simulink model "adsl_sim"  (Simulink 6.0)
settings: Solver=ode45  SolverMode=SingleTasking  StartTime=0.0  StopTime=2  RelTol=1e-3
PreLoadFcn:
  | % variables are initialized through the Model Workspace
model workspace: external: M-Code (data not in the file)
values from neighbouring files (symbols this model uses):
  H = conv2(chCoeff',W)    [eq_computecostfcn.m]    (also in eq_costfcnconverg.m = conv2(eq.chCoeff,W))
undefined symbols (not defined in the file or in its folder): b, rsgenpoly, slcm
libraries: commdigbbndam2 x512, simulink x37, commutil2 x8, commblkcod2 x4, commsequence2 x4, commsink2 x4, commcrc2 x4, commcnvintrlv2 x2, dspxfrm3 x2, dspsrcs4 x2, dspsigattribs x1, dspmtrx3 x1
(part 2 of 5)

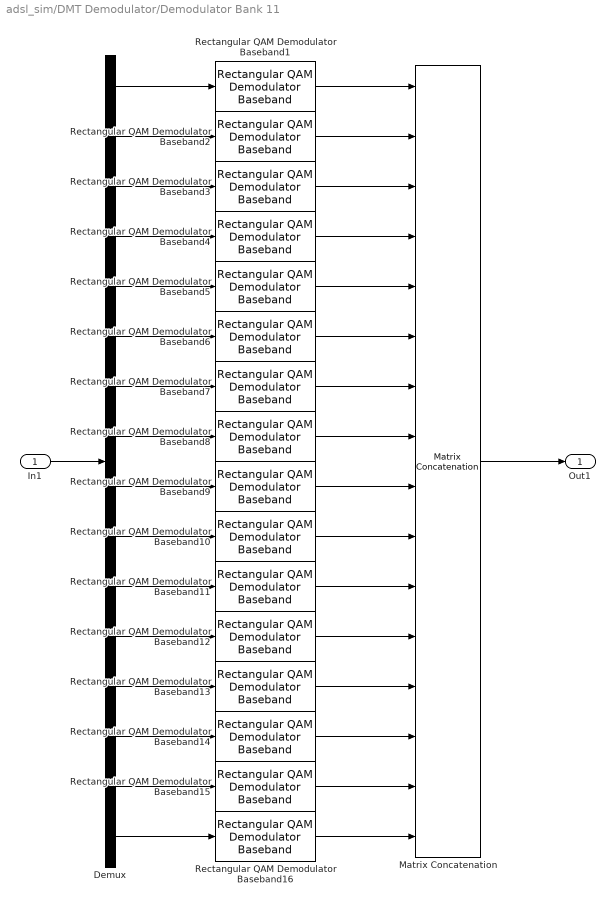
== system adsl_sim/DMT Demodulator/Demodulator Bank 11 ==
  In1 : Inport  LatchInput=off
  Demux : Demux  Outputs=16
  Matrix Concatenation : simulink/Math Operations/Matrix Concatenation  numInports=16  catMethod=Vertical
  Rectangular QAM Demodulator Baseband1 : commdigbbndam2/Rectangular QAM Demodulator Baseband  M=2^b(offset+1)  OutType=Bit  Dec=Gray  PowType=Average Power  MinDist=2  AvgPow=1  PeakPow=1  Ph=0  numSamp=1
  Rectangular QAM Demodulator Baseband10 : commdigbbndam2/Rectangular QAM Demodulator Baseband  M=2^b(offset+10)  OutType=Bit  Dec=Gray  PowType=Average Power  MinDist=2  AvgPow=1  PeakPow=1  Ph=0  numSamp=1
  Rectangular QAM Demodulator Baseband11 : commdigbbndam2/Rectangular QAM Demodulator Baseband  M=2^b(offset+11)  OutType=Bit  Dec=Gray  PowType=Average Power  MinDist=2  AvgPow=1  PeakPow=1  Ph=0  numSamp=1
  Rectangular QAM Demodulator Baseband12 : commdigbbndam2/Rectangular QAM Demodulator Baseband  M=2^b(offset+12)  OutType=Bit  Dec=Gray  PowType=Average Power  MinDist=2  AvgPow=1  PeakPow=1  Ph=0  numSamp=1
  Rectangular QAM Demodulator Baseband13 : commdigbbndam2/Rectangular QAM Demodulator Baseband  M=2^b(offset+13)  OutType=Bit  Dec=Gray  PowType=Average Power  MinDist=2  AvgPow=1  PeakPow=1  Ph=0  numSamp=1
  Rectangular QAM Demodulator Baseband14 : commdigbbndam2/Rectangular QAM Demodulator Baseband  M=2^b(offset+14)  OutType=Bit  Dec=Gray  PowType=Average Power  MinDist=2  AvgPow=1  PeakPow=1  Ph=0  numSamp=1
  Rectangular QAM Demodulator Baseband15 : commdigbbndam2/Rectangular QAM Demodulator Baseband  M=2^b(offset+15)  OutType=Bit  Dec=Gray  PowType=Average Power  MinDist=2  AvgPow=1  PeakPow=1  Ph=0  numSamp=1
  Rectangular QAM Demodulator Baseband16 : commdigbbndam2/Rectangular QAM Demodulator Baseband  M=2^b(offset+16)  OutType=Bit  Dec=Gray  PowType=Average Power  MinDist=2  AvgPow=1  PeakPow=1  Ph=0  numSamp=1
  Rectangular QAM Demodulator Baseband2 : commdigbbndam2/Rectangular QAM Demodulator Baseband  M=2^b(offset+2)  OutType=Bit  Dec=Gray  PowType=Average Power  MinDist=2  AvgPow=1  PeakPow=1  Ph=0  numSamp=1
  Rectangular QAM Demodulator Baseband3 : commdigbbndam2/Rectangular QAM Demodulator Baseband  M=2^b(offset+3)  OutType=Bit  Dec=Gray  PowType=Average Power  MinDist=2  AvgPow=1  PeakPow=1  Ph=0  numSamp=1
  Rectangular QAM Demodulator Baseband4 : commdigbbndam2/Rectangular QAM Demodulator Baseband  M=2^b(offset+4)  OutType=Bit  Dec=Gray  PowType=Average Power  MinDist=2  AvgPow=1  PeakPow=1  Ph=0  numSamp=1
  Rectangular QAM Demodulator Baseband5 : commdigbbndam2/Rectangular QAM Demodulator Baseband  M=2^b(offset+5)  OutType=Bit  Dec=Gray  PowType=Average Power  MinDist=2  AvgPow=1  PeakPow=1  Ph=0  numSamp=1
  Rectangular QAM Demodulator Baseband6 : commdigbbndam2/Rectangular QAM Demodulator Baseband  M=2^b(offset+6)  OutType=Bit  Dec=Gray  PowType=Average Power  MinDist=2  AvgPow=1  PeakPow=1  Ph=0  numSamp=1
  Rectangular QAM Demodulator Baseband7 : commdigbbndam2/Rectangular QAM Demodulator Baseband  M=2^b(offset+7)  OutType=Bit  Dec=Gray  PowType=Average Power  MinDist=2  AvgPow=1  PeakPow=1  Ph=0  numSamp=1
  Rectangular QAM Demodulator Baseband8 : commdigbbndam2/Rectangular QAM Demodulator Baseband  M=2^b(offset+8)  OutType=Bit  Dec=Gray  PowType=Average Power  MinDist=2  AvgPow=1  PeakPow=1  Ph=0  numSamp=1
  Rectangular QAM Demodulator Baseband9 : commdigbbndam2/Rectangular QAM Demodulator Baseband  M=2^b(offset+9)  OutType=Bit  Dec=Gray  PowType=Average Power  MinDist=2  AvgPow=1  PeakPow=1  Ph=0  numSamp=1
  Out1 : Outport
  wires:
  In1/1 -> Demux/1
  Matrix Concatenation/1 -> Out1/1
  Demux/16 -> Rectangular QAM Demodulator Baseband16/1
  Demux/15 -> Rectangular QAM Demodulator Baseband15/1
  Demux/14 -> Rectangular QAM Demodulator Baseband14/1
  Demux/13 -> Rectangular QAM Demodulator Baseband13/1
  Demux/12 -> Rectangular QAM Demodulator Baseband12/1
  Demux/11 -> Rectangular QAM Demodulator Baseband11/1
  Demux/10 -> Rectangular QAM Demodulator Baseband10/1
  Demux/9 -> Rectangular QAM Demodulator Baseband9/1
  Demux/8 -> Rectangular QAM Demodulator Baseband8/1
  Demux/7 -> Rectangular QAM Demodulator Baseband7/1
  Demux/6 -> Rectangular QAM Demodulator Baseband6/1
  Demux/5 -> Rectangular QAM Demodulator Baseband5/1
  Demux/4 -> Rectangular QAM Demodulator Baseband4/1
  Demux/3 -> Rectangular QAM Demodulator Baseband3/1
  Demux/2 -> Rectangular QAM Demodulator Baseband2/1
  Demux/1 -> Rectangular QAM Demodulator Baseband1/1
  Rectangular QAM Demodulator Baseband16/1 -> Matrix Concatenation/16
  Rectangular QAM Demodulator Baseband15/1 -> Matrix Concatenation/15
  Rectangular QAM Demodulator Baseband14/1 -> Matrix Concatenation/14
  Rectangular QAM Demodulator Baseband13/1 -> Matrix Concatenation/13
  Rectangular QAM Demodulator Baseband12/1 -> Matrix Concatenation/12
  Rectangular QAM Demodulator Baseband11/1 -> Matrix Concatenation/11
  Rectangular QAM Demodulator Baseband10/1 -> Matrix Concatenation/10
  Rectangular QAM Demodulator Baseband9/1 -> Matrix Concatenation/9
  Rectangular QAM Demodulator Baseband8/1 -> Matrix Concatenation/8
  Rectangular QAM Demodulator Baseband7/1 -> Matrix Concatenation/7
  Rectangular QAM Demodulator Baseband6/1 -> Matrix Concatenation/6
  Rectangular QAM Demodulator Baseband5/1 -> Matrix Concatenation/5
  Rectangular QAM Demodulator Baseband4/1 -> Matrix Concatenation/4
  Rectangular QAM Demodulator Baseband3/1 -> Matrix Concatenation/3
  Rectangular QAM Demodulator Baseband2/1 -> Matrix Concatenation/2
  Rectangular QAM Demodulator Baseband1/1 -> Matrix Concatenation/1

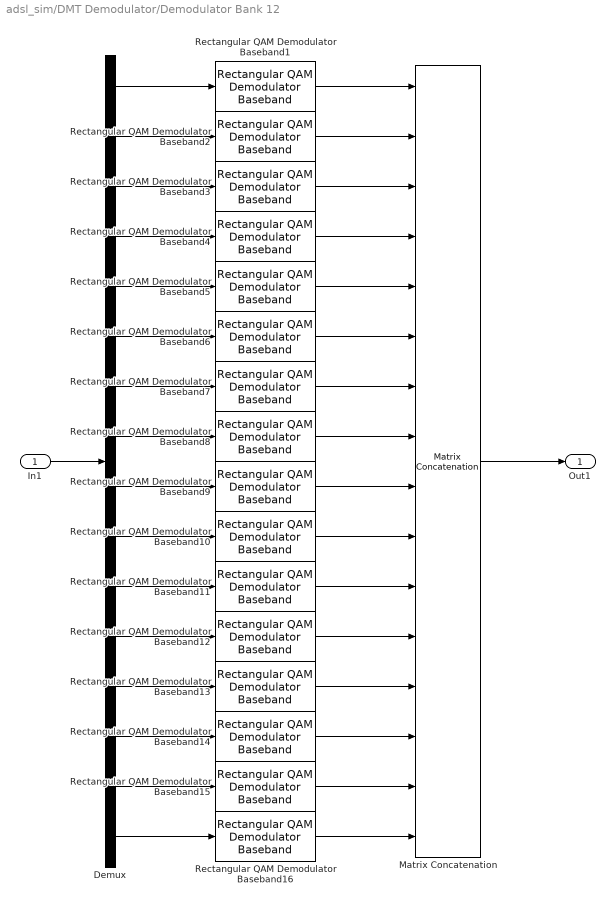
== system adsl_sim/DMT Demodulator/Demodulator Bank 12 ==
  In1 : Inport  LatchInput=off
  Demux : Demux  Outputs=16
  Matrix Concatenation : simulink/Math Operations/Matrix Concatenation  numInports=16  catMethod=Vertical
  Rectangular QAM Demodulator Baseband1 : commdigbbndam2/Rectangular QAM Demodulator Baseband  M=2^b(offset+1)  OutType=Bit  Dec=Gray  PowType=Average Power  MinDist=2  AvgPow=1  PeakPow=1  Ph=0  numSamp=1
  Rectangular QAM Demodulator Baseband10 : commdigbbndam2/Rectangular QAM Demodulator Baseband  M=2^b(offset+10)  OutType=Bit  Dec=Gray  PowType=Average Power  MinDist=2  AvgPow=1  PeakPow=1  Ph=0  numSamp=1
  Rectangular QAM Demodulator Baseband11 : commdigbbndam2/Rectangular QAM Demodulator Baseband  M=2^b(offset+11)  OutType=Bit  Dec=Gray  PowType=Average Power  MinDist=2  AvgPow=1  PeakPow=1  Ph=0  numSamp=1
  Rectangular QAM Demodulator Baseband12 : commdigbbndam2/Rectangular QAM Demodulator Baseband  M=2^b(offset+12)  OutType=Bit  Dec=Gray  PowType=Average Power  MinDist=2  AvgPow=1  PeakPow=1  Ph=0  numSamp=1
  Rectangular QAM Demodulator Baseband13 : commdigbbndam2/Rectangular QAM Demodulator Baseband  M=2^b(offset+13)  OutType=Bit  Dec=Gray  PowType=Average Power  MinDist=2  AvgPow=1  PeakPow=1  Ph=0  numSamp=1
  Rectangular QAM Demodulator Baseband14 : commdigbbndam2/Rectangular QAM Demodulator Baseband  M=2^b(offset+14)  OutType=Bit  Dec=Gray  PowType=Average Power  MinDist=2  AvgPow=1  PeakPow=1  Ph=0  numSamp=1
  Rectangular QAM Demodulator Baseband15 : commdigbbndam2/Rectangular QAM Demodulator Baseband  M=2^b(offset+15)  OutType=Bit  Dec=Gray  PowType=Average Power  MinDist=2  AvgPow=1  PeakPow=1  Ph=0  numSamp=1
  Rectangular QAM Demodulator Baseband16 : commdigbbndam2/Rectangular QAM Demodulator Baseband  M=2^b(offset+16)  OutType=Bit  Dec=Gray  PowType=Average Power  MinDist=2  AvgPow=1  PeakPow=1  Ph=0  numSamp=1
  Rectangular QAM Demodulator Baseband2 : commdigbbndam2/Rectangular QAM Demodulator Baseband  M=2^b(offset+2)  OutType=Bit  Dec=Gray  PowType=Average Power  MinDist=2  AvgPow=1  PeakPow=1  Ph=0  numSamp=1
  Rectangular QAM Demodulator Baseband3 : commdigbbndam2/Rectangular QAM Demodulator Baseband  M=2^b(offset+3)  OutType=Bit  Dec=Gray  PowType=Average Power  MinDist=2  AvgPow=1  PeakPow=1  Ph=0  numSamp=1
  Rectangular QAM Demodulator Baseband4 : commdigbbndam2/Rectangular QAM Demodulator Baseband  M=2^b(offset+4)  OutType=Bit  Dec=Gray  PowType=Average Power  MinDist=2  AvgPow=1  PeakPow=1  Ph=0  numSamp=1
  Rectangular QAM Demodulator Baseband5 : commdigbbndam2/Rectangular QAM Demodulator Baseband  M=2^b(offset+5)  OutType=Bit  Dec=Gray  PowType=Average Power  MinDist=2  AvgPow=1  PeakPow=1  Ph=0  numSamp=1
  Rectangular QAM Demodulator Baseband6 : commdigbbndam2/Rectangular QAM Demodulator Baseband  M=2^b(offset+6)  OutType=Bit  Dec=Gray  PowType=Average Power  MinDist=2  AvgPow=1  PeakPow=1  Ph=0  numSamp=1
  Rectangular QAM Demodulator Baseband7 : commdigbbndam2/Rectangular QAM Demodulator Baseband  M=2^b(offset+7)  OutType=Bit  Dec=Gray  PowType=Average Power  MinDist=2  AvgPow=1  PeakPow=1  Ph=0  numSamp=1
  Rectangular QAM Demodulator Baseband8 : commdigbbndam2/Rectangular QAM Demodulator Baseband  M=2^b(offset+8)  OutType=Bit  Dec=Gray  PowType=Average Power  MinDist=2  AvgPow=1  PeakPow=1  Ph=0  numSamp=1
  Rectangular QAM Demodulator Baseband9 : commdigbbndam2/Rectangular QAM Demodulator Baseband  M=2^b(offset+9)  OutType=Bit  Dec=Gray  PowType=Average Power  MinDist=2  AvgPow=1  PeakPow=1  Ph=0  numSamp=1
  Out1 : Outport
  wires:
  Rectangular QAM Demodulator Baseband1/1 -> Matrix Concatenation/1
  Rectangular QAM Demodulator Baseband2/1 -> Matrix Concatenation/2
  Rectangular QAM Demodulator Baseband3/1 -> Matrix Concatenation/3
  Rectangular QAM Demodulator Baseband4/1 -> Matrix Concatenation/4
  Rectangular QAM Demodulator Baseband5/1 -> Matrix Concatenation/5
  Rectangular QAM Demodulator Baseband6/1 -> Matrix Concatenation/6
  Rectangular QAM Demodulator Baseband7/1 -> Matrix Concatenation/7
  Rectangular QAM Demodulator Baseband8/1 -> Matrix Concatenation/8
  Rectangular QAM Demodulator Baseband9/1 -> Matrix Concatenation/9
  Rectangular QAM Demodulator Baseband10/1 -> Matrix Concatenation/10
  Rectangular QAM Demodulator Baseband11/1 -> Matrix Concatenation/11
  Rectangular QAM Demodulator Baseband12/1 -> Matrix Concatenation/12
  Rectangular QAM Demodulator Baseband13/1 -> Matrix Concatenation/13
  Rectangular QAM Demodulator Baseband14/1 -> Matrix Concatenation/14
  Rectangular QAM Demodulator Baseband15/1 -> Matrix Concatenation/15
  Rectangular QAM Demodulator Baseband16/1 -> Matrix Concatenation/16
  Demux/1 -> Rectangular QAM Demodulator Baseband1/1
  Demux/2 -> Rectangular QAM Demodulator Baseband2/1
  Demux/3 -> Rectangular QAM Demodulator Baseband3/1
  Demux/4 -> Rectangular QAM Demodulator Baseband4/1
  Demux/5 -> Rectangular QAM Demodulator Baseband5/1
  Demux/6 -> Rectangular QAM Demodulator Baseband6/1
  Demux/7 -> Rectangular QAM Demodulator Baseband7/1
  Demux/8 -> Rectangular QAM Demodulator Baseband8/1
  Demux/9 -> Rectangular QAM Demodulator Baseband9/1
  Demux/10 -> Rectangular QAM Demodulator Baseband10/1
  Demux/11 -> Rectangular QAM Demodulator Baseband11/1
  Demux/12 -> Rectangular QAM Demodulator Baseband12/1
  Demux/13 -> Rectangular QAM Demodulator Baseband13/1
  Demux/14 -> Rectangular QAM Demodulator Baseband14/1
  Demux/15 -> Rectangular QAM Demodulator Baseband15/1
  Demux/16 -> Rectangular QAM Demodulator Baseband16/1
  Matrix Concatenation/1 -> Out1/1
  In1/1 -> Demux/1

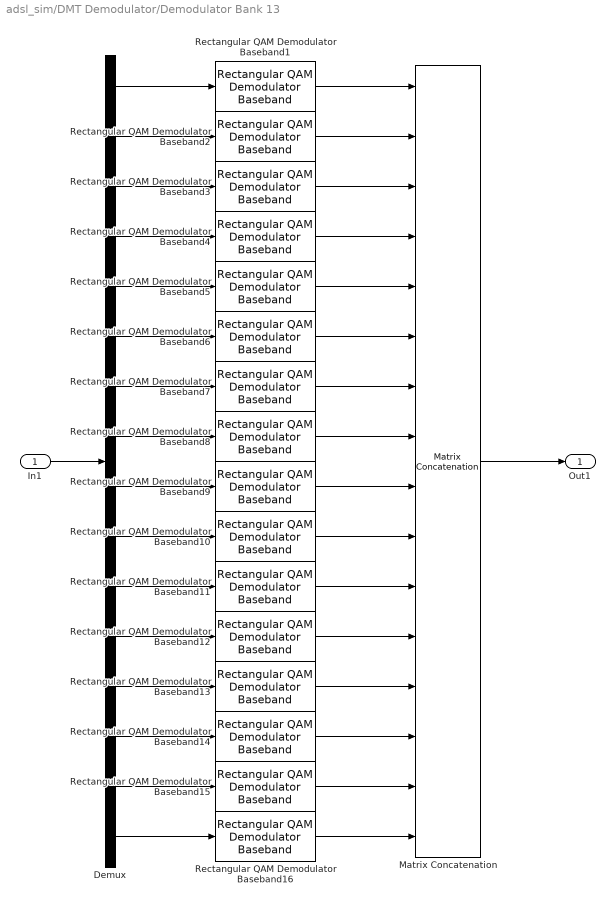
== system adsl_sim/DMT Demodulator/Demodulator Bank 13 ==
  In1 : Inport  LatchInput=off
  Demux : Demux  Outputs=16
  Matrix Concatenation : simulink/Math Operations/Matrix Concatenation  numInports=16  catMethod=Vertical
  Rectangular QAM Demodulator Baseband1 : commdigbbndam2/Rectangular QAM Demodulator Baseband  M=2^b(offset+1)  OutType=Bit  Dec=Gray  PowType=Average Power  MinDist=2  AvgPow=1  PeakPow=1  Ph=0  numSamp=1
  Rectangular QAM Demodulator Baseband10 : commdigbbndam2/Rectangular QAM Demodulator Baseband  M=2^b(offset+10)  OutType=Bit  Dec=Gray  PowType=Average Power  MinDist=2  AvgPow=1  PeakPow=1  Ph=0  numSamp=1
  Rectangular QAM Demodulator Baseband11 : commdigbbndam2/Rectangular QAM Demodulator Baseband  M=2^b(offset+11)  OutType=Bit  Dec=Gray  PowType=Average Power  MinDist=2  AvgPow=1  PeakPow=1  Ph=0  numSamp=1
  Rectangular QAM Demodulator Baseband12 : commdigbbndam2/Rectangular QAM Demodulator Baseband  M=2^b(offset+12)  OutType=Bit  Dec=Gray  PowType=Average Power  MinDist=2  AvgPow=1  PeakPow=1  Ph=0  numSamp=1
  Rectangular QAM Demodulator Baseband13 : commdigbbndam2/Rectangular QAM Demodulator Baseband  M=2^b(offset+13)  OutType=Bit  Dec=Gray  PowType=Average Power  MinDist=2  AvgPow=1  PeakPow=1  Ph=0  numSamp=1
  Rectangular QAM Demodulator Baseband14 : commdigbbndam2/Rectangular QAM Demodulator Baseband  M=2^b(offset+14)  OutType=Bit  Dec=Gray  PowType=Average Power  MinDist=2  AvgPow=1  PeakPow=1  Ph=0  numSamp=1
  Rectangular QAM Demodulator Baseband15 : commdigbbndam2/Rectangular QAM Demodulator Baseband  M=2^b(offset+15)  OutType=Bit  Dec=Gray  PowType=Average Power  MinDist=2  AvgPow=1  PeakPow=1  Ph=0  numSamp=1
  Rectangular QAM Demodulator Baseband16 : commdigbbndam2/Rectangular QAM Demodulator Baseband  M=2^b(offset+16)  OutType=Bit  Dec=Gray  PowType=Average Power  MinDist=2  AvgPow=1  PeakPow=1  Ph=0  numSamp=1
  Rectangular QAM Demodulator Baseband2 : commdigbbndam2/Rectangular QAM Demodulator Baseband  M=2^b(offset+2)  OutType=Bit  Dec=Gray  PowType=Average Power  MinDist=2  AvgPow=1  PeakPow=1  Ph=0  numSamp=1
  Rectangular QAM Demodulator Baseband3 : commdigbbndam2/Rectangular QAM Demodulator Baseband  M=2^b(offset+3)  OutType=Bit  Dec=Gray  PowType=Average Power  MinDist=2  AvgPow=1  PeakPow=1  Ph=0  numSamp=1
  Rectangular QAM Demodulator Baseband4 : commdigbbndam2/Rectangular QAM Demodulator Baseband  M=2^b(offset+4)  OutType=Bit  Dec=Gray  PowType=Average Power  MinDist=2  AvgPow=1  PeakPow=1  Ph=0  numSamp=1
  Rectangular QAM Demodulator Baseband5 : commdigbbndam2/Rectangular QAM Demodulator Baseband  M=2^b(offset+5)  OutType=Bit  Dec=Gray  PowType=Average Power  MinDist=2  AvgPow=1  PeakPow=1  Ph=0  numSamp=1
  Rectangular QAM Demodulator Baseband6 : commdigbbndam2/Rectangular QAM Demodulator Baseband  M=2^b(offset+6)  OutType=Bit  Dec=Gray  PowType=Average Power  MinDist=2  AvgPow=1  PeakPow=1  Ph=0  numSamp=1
  Rectangular QAM Demodulator Baseband7 : commdigbbndam2/Rectangular QAM Demodulator Baseband  M=2^b(offset+7)  OutType=Bit  Dec=Gray  PowType=Average Power  MinDist=2  AvgPow=1  PeakPow=1  Ph=0  numSamp=1
  Rectangular QAM Demodulator Baseband8 : commdigbbndam2/Rectangular QAM Demodulator Baseband  M=2^b(offset+8)  OutType=Bit  Dec=Gray  PowType=Average Power  MinDist=2  AvgPow=1  PeakPow=1  Ph=0  numSamp=1
  Rectangular QAM Demodulator Baseband9 : commdigbbndam2/Rectangular QAM Demodulator Baseband  M=2^b(offset+9)  OutType=Bit  Dec=Gray  PowType=Average Power  MinDist=2  AvgPow=1  PeakPow=1  Ph=0  numSamp=1
  Out1 : Outport
  wires:
  In1/1 -> Demux/1
  Matrix Concatenation/1 -> Out1/1
  Demux/16 -> Rectangular QAM Demodulator Baseband16/1
  Demux/15 -> Rectangular QAM Demodulator Baseband15/1
  Demux/14 -> Rectangular QAM Demodulator Baseband14/1
  Demux/13 -> Rectangular QAM Demodulator Baseband13/1
  Demux/12 -> Rectangular QAM Demodulator Baseband12/1
  Demux/11 -> Rectangular QAM Demodulator Baseband11/1
  Demux/10 -> Rectangular QAM Demodulator Baseband10/1
  Demux/9 -> Rectangular QAM Demodulator Baseband9/1
  Demux/8 -> Rectangular QAM Demodulator Baseband8/1
  Demux/7 -> Rectangular QAM Demodulator Baseband7/1
  Demux/6 -> Rectangular QAM Demodulator Baseband6/1
  Demux/5 -> Rectangular QAM Demodulator Baseband5/1
  Demux/4 -> Rectangular QAM Demodulator Baseband4/1
  Demux/3 -> Rectangular QAM Demodulator Baseband3/1
  Demux/2 -> Rectangular QAM Demodulator Baseband2/1
  Demux/1 -> Rectangular QAM Demodulator Baseband1/1
  Rectangular QAM Demodulator Baseband16/1 -> Matrix Concatenation/16
  Rectangular QAM Demodulator Baseband15/1 -> Matrix Concatenation/15
  Rectangular QAM Demodulator Baseband14/1 -> Matrix Concatenation/14
  Rectangular QAM Demodulator Baseband13/1 -> Matrix Concatenation/13
  Rectangular QAM Demodulator Baseband12/1 -> Matrix Concatenation/12
  Rectangular QAM Demodulator Baseband11/1 -> Matrix Concatenation/11
  Rectangular QAM Demodulator Baseband10/1 -> Matrix Concatenation/10
  Rectangular QAM Demodulator Baseband9/1 -> Matrix Concatenation/9
  Rectangular QAM Demodulator Baseband8/1 -> Matrix Concatenation/8
  Rectangular QAM Demodulator Baseband7/1 -> Matrix Concatenation/7
  Rectangular QAM Demodulator Baseband6/1 -> Matrix Concatenation/6
  Rectangular QAM Demodulator Baseband5/1 -> Matrix Concatenation/5
  Rectangular QAM Demodulator Baseband4/1 -> Matrix Concatenation/4
  Rectangular QAM Demodulator Baseband3/1 -> Matrix Concatenation/3
  Rectangular QAM Demodulator Baseband2/1 -> Matrix Concatenation/2
  Rectangular QAM Demodulator Baseband1/1 -> Matrix Concatenation/1

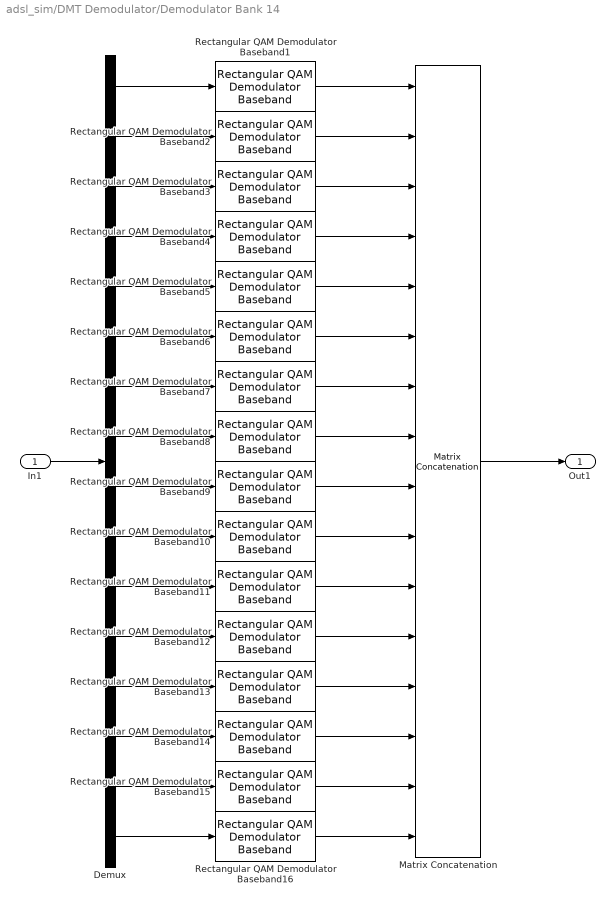
== system adsl_sim/DMT Demodulator/Demodulator Bank 14 ==
  In1 : Inport  LatchInput=off
  Demux : Demux  Outputs=16
  Matrix Concatenation : simulink/Math Operations/Matrix Concatenation  numInports=16  catMethod=Vertical
  Rectangular QAM Demodulator Baseband1 : commdigbbndam2/Rectangular QAM Demodulator Baseband  M=2^b(offset+1)  OutType=Bit  Dec=Gray  PowType=Average Power  MinDist=2  AvgPow=1  PeakPow=1  Ph=0  numSamp=1
  Rectangular QAM Demodulator Baseband10 : commdigbbndam2/Rectangular QAM Demodulator Baseband  M=2^b(offset+10)  OutType=Bit  Dec=Gray  PowType=Average Power  MinDist=2  AvgPow=1  PeakPow=1  Ph=0  numSamp=1
  Rectangular QAM Demodulator Baseband11 : commdigbbndam2/Rectangular QAM Demodulator Baseband  M=2^b(offset+11)  OutType=Bit  Dec=Gray  PowType=Average Power  MinDist=2  AvgPow=1  PeakPow=1  Ph=0  numSamp=1
  Rectangular QAM Demodulator Baseband12 : commdigbbndam2/Rectangular QAM Demodulator Baseband  M=2^b(offset+12)  OutType=Bit  Dec=Gray  PowType=Average Power  MinDist=2  AvgPow=1  PeakPow=1  Ph=0  numSamp=1
  Rectangular QAM Demodulator Baseband13 : commdigbbndam2/Rectangular QAM Demodulator Baseband  M=2^b(offset+13)  OutType=Bit  Dec=Gray  PowType=Average Power  MinDist=2  AvgPow=1  PeakPow=1  Ph=0  numSamp=1
  Rectangular QAM Demodulator Baseband14 : commdigbbndam2/Rectangular QAM Demodulator Baseband  M=2^b(offset+14)  OutType=Bit  Dec=Gray  PowType=Average Power  MinDist=2  AvgPow=1  PeakPow=1  Ph=0  numSamp=1
  Rectangular QAM Demodulator Baseband15 : commdigbbndam2/Rectangular QAM Demodulator Baseband  M=2^b(offset+15)  OutType=Bit  Dec=Gray  PowType=Average Power  MinDist=2  AvgPow=1  PeakPow=1  Ph=0  numSamp=1
  Rectangular QAM Demodulator Baseband16 : commdigbbndam2/Rectangular QAM Demodulator Baseband  M=2^b(offset+16)  OutType=Bit  Dec=Gray  PowType=Average Power  MinDist=2  AvgPow=1  PeakPow=1  Ph=0  numSamp=1
  Rectangular QAM Demodulator Baseband2 : commdigbbndam2/Rectangular QAM Demodulator Baseband  M=2^b(offset+2)  OutType=Bit  Dec=Gray  PowType=Average Power  MinDist=2  AvgPow=1  PeakPow=1  Ph=0  numSamp=1
  Rectangular QAM Demodulator Baseband3 : commdigbbndam2/Rectangular QAM Demodulator Baseband  M=2^b(offset+3)  OutType=Bit  Dec=Gray  PowType=Average Power  MinDist=2  AvgPow=1  PeakPow=1  Ph=0  numSamp=1
  Rectangular QAM Demodulator Baseband4 : commdigbbndam2/Rectangular QAM Demodulator Baseband  M=2^b(offset+4)  OutType=Bit  Dec=Gray  PowType=Average Power  MinDist=2  AvgPow=1  PeakPow=1  Ph=0  numSamp=1
  Rectangular QAM Demodulator Baseband5 : commdigbbndam2/Rectangular QAM Demodulator Baseband  M=2^b(offset+5)  OutType=Bit  Dec=Gray  PowType=Average Power  MinDist=2  AvgPow=1  PeakPow=1  Ph=0  numSamp=1
  Rectangular QAM Demodulator Baseband6 : commdigbbndam2/Rectangular QAM Demodulator Baseband  M=2^b(offset+6)  OutType=Bit  Dec=Gray  PowType=Average Power  MinDist=2  AvgPow=1  PeakPow=1  Ph=0  numSamp=1
  Rectangular QAM Demodulator Baseband7 : commdigbbndam2/Rectangular QAM Demodulator Baseband  M=2^b(offset+7)  OutType=Bit  Dec=Gray  PowType=Average Power  MinDist=2  AvgPow=1  PeakPow=1  Ph=0  numSamp=1
  Rectangular QAM Demodulator Baseband8 : commdigbbndam2/Rectangular QAM Demodulator Baseband  M=2^b(offset+8)  OutType=Bit  Dec=Gray  PowType=Average Power  MinDist=2  AvgPow=1  PeakPow=1  Ph=0  numSamp=1
  Rectangular QAM Demodulator Baseband9 : commdigbbndam2/Rectangular QAM Demodulator Baseband  M=2^b(offset+9)  OutType=Bit  Dec=Gray  PowType=Average Power  MinDist=2  AvgPow=1  PeakPow=1  Ph=0  numSamp=1
  Out1 : Outport
  wires:
  Rectangular QAM Demodulator Baseband1/1 -> Matrix Concatenation/1
  Rectangular QAM Demodulator Baseband2/1 -> Matrix Concatenation/2
  Rectangular QAM Demodulator Baseband3/1 -> Matrix Concatenation/3
  Rectangular QAM Demodulator Baseband4/1 -> Matrix Concatenation/4
  Rectangular QAM Demodulator Baseband5/1 -> Matrix Concatenation/5
  Rectangular QAM Demodulator Baseband6/1 -> Matrix Concatenation/6
  Rectangular QAM Demodulator Baseband7/1 -> Matrix Concatenation/7
  Rectangular QAM Demodulator Baseband8/1 -> Matrix Concatenation/8
  Rectangular QAM Demodulator Baseband9/1 -> Matrix Concatenation/9
  Rectangular QAM Demodulator Baseband10/1 -> Matrix Concatenation/10
  Rectangular QAM Demodulator Baseband11/1 -> Matrix Concatenation/11
  Rectangular QAM Demodulator Baseband12/1 -> Matrix Concatenation/12
  Rectangular QAM Demodulator Baseband13/1 -> Matrix Concatenation/13
  Rectangular QAM Demodulator Baseband14/1 -> Matrix Concatenation/14
  Rectangular QAM Demodulator Baseband15/1 -> Matrix Concatenation/15
  Rectangular QAM Demodulator Baseband16/1 -> Matrix Concatenation/16
  Demux/1 -> Rectangular QAM Demodulator Baseband1/1
  Demux/2 -> Rectangular QAM Demodulator Baseband2/1
  Demux/3 -> Rectangular QAM Demodulator Baseband3/1
  Demux/4 -> Rectangular QAM Demodulator Baseband4/1
  Demux/5 -> Rectangular QAM Demodulator Baseband5/1
  Demux/6 -> Rectangular QAM Demodulator Baseband6/1
  Demux/7 -> Rectangular QAM Demodulator Baseband7/1
  Demux/8 -> Rectangular QAM Demodulator Baseband8/1
  Demux/9 -> Rectangular QAM Demodulator Baseband9/1
  Demux/10 -> Rectangular QAM Demodulator Baseband10/1
  Demux/11 -> Rectangular QAM Demodulator Baseband11/1
  Demux/12 -> Rectangular QAM Demodulator Baseband12/1
  Demux/13 -> Rectangular QAM Demodulator Baseband13/1
  Demux/14 -> Rectangular QAM Demodulator Baseband14/1
  Demux/15 -> Rectangular QAM Demodulator Baseband15/1
  Demux/16 -> Rectangular QAM Demodulator Baseband16/1
  Matrix Concatenation/1 -> Out1/1
  In1/1 -> Demux/1

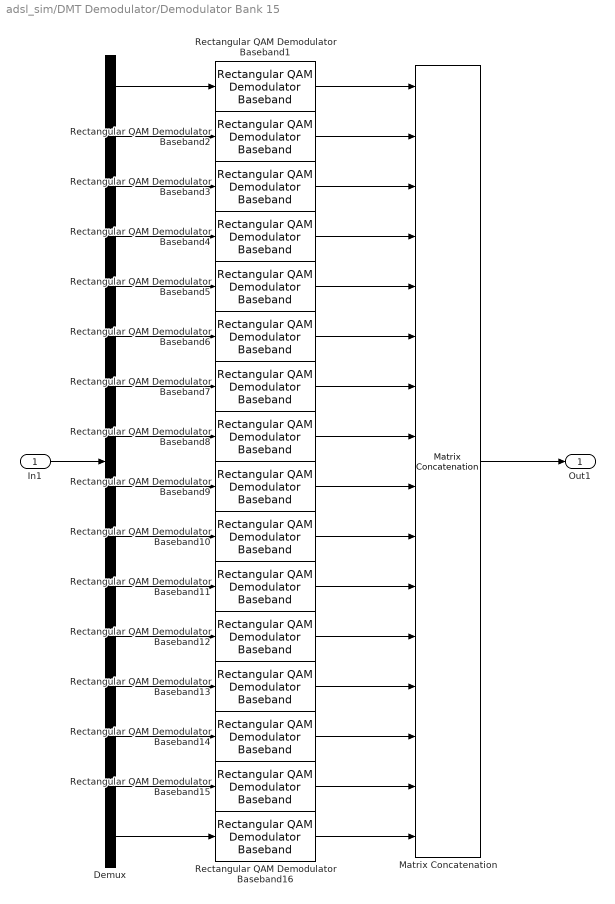
== system adsl_sim/DMT Demodulator/Demodulator Bank 15 ==
  In1 : Inport  LatchInput=off
  Demux : Demux  Outputs=16
  Matrix Concatenation : simulink/Math Operations/Matrix Concatenation  numInports=16  catMethod=Vertical
  Rectangular QAM Demodulator Baseband1 : commdigbbndam2/Rectangular QAM Demodulator Baseband  M=2^b(offset+1)  OutType=Bit  Dec=Gray  PowType=Average Power  MinDist=2  AvgPow=1  PeakPow=1  Ph=0  numSamp=1
  Rectangular QAM Demodulator Baseband10 : commdigbbndam2/Rectangular QAM Demodulator Baseband  M=2^b(offset+10)  OutType=Bit  Dec=Gray  PowType=Average Power  MinDist=2  AvgPow=1  PeakPow=1  Ph=0  numSamp=1
  Rectangular QAM Demodulator Baseband11 : commdigbbndam2/Rectangular QAM Demodulator Baseband  M=2^b(offset+11)  OutType=Bit  Dec=Gray  PowType=Average Power  MinDist=2  AvgPow=1  PeakPow=1  Ph=0  numSamp=1
  Rectangular QAM Demodulator Baseband12 : commdigbbndam2/Rectangular QAM Demodulator Baseband  M=2^b(offset+12)  OutType=Bit  Dec=Gray  PowType=Average Power  MinDist=2  AvgPow=1  PeakPow=1  Ph=0  numSamp=1
  Rectangular QAM Demodulator Baseband13 : commdigbbndam2/Rectangular QAM Demodulator Baseband  M=2^b(offset+13)  OutType=Bit  Dec=Gray  PowType=Average Power  MinDist=2  AvgPow=1  PeakPow=1  Ph=0  numSamp=1
  Rectangular QAM Demodulator Baseband14 : commdigbbndam2/Rectangular QAM Demodulator Baseband  M=2^b(offset+14)  OutType=Bit  Dec=Gray  PowType=Average Power  MinDist=2  AvgPow=1  PeakPow=1  Ph=0  numSamp=1
  Rectangular QAM Demodulator Baseband15 : commdigbbndam2/Rectangular QAM Demodulator Baseband  M=2^b(offset+15)  OutType=Bit  Dec=Gray  PowType=Average Power  MinDist=2  AvgPow=1  PeakPow=1  Ph=0  numSamp=1
  Rectangular QAM Demodulator Baseband16 : commdigbbndam2/Rectangular QAM Demodulator Baseband  M=2^b(offset+16)  OutType=Bit  Dec=Gray  PowType=Average Power  MinDist=2  AvgPow=1  PeakPow=1  Ph=0  numSamp=1
  Rectangular QAM Demodulator Baseband2 : commdigbbndam2/Rectangular QAM Demodulator Baseband  M=2^b(offset+2)  OutType=Bit  Dec=Gray  PowType=Average Power  MinDist=2  AvgPow=1  PeakPow=1  Ph=0  numSamp=1
  Rectangular QAM Demodulator Baseband3 : commdigbbndam2/Rectangular QAM Demodulator Baseband  M=2^b(offset+3)  OutType=Bit  Dec=Gray  PowType=Average Power  MinDist=2  AvgPow=1  PeakPow=1  Ph=0  numSamp=1
  Rectangular QAM Demodulator Baseband4 : commdigbbndam2/Rectangular QAM Demodulator Baseband  M=2^b(offset+4)  OutType=Bit  Dec=Gray  PowType=Average Power  MinDist=2  AvgPow=1  PeakPow=1  Ph=0  numSamp=1
  Rectangular QAM Demodulator Baseband5 : commdigbbndam2/Rectangular QAM Demodulator Baseband  M=2^b(offset+5)  OutType=Bit  Dec=Gray  PowType=Average Power  MinDist=2  AvgPow=1  PeakPow=1  Ph=0  numSamp=1
  Rectangular QAM Demodulator Baseband6 : commdigbbndam2/Rectangular QAM Demodulator Baseband  M=2^b(offset+6)  OutType=Bit  Dec=Gray  PowType=Average Power  MinDist=2  AvgPow=1  PeakPow=1  Ph=0  numSamp=1
  Rectangular QAM Demodulator Baseband7 : commdigbbndam2/Rectangular QAM Demodulator Baseband  M=2^b(offset+7)  OutType=Bit  Dec=Gray  PowType=Average Power  MinDist=2  AvgPow=1  PeakPow=1  Ph=0  numSamp=1
  Rectangular QAM Demodulator Baseband8 : commdigbbndam2/Rectangular QAM Demodulator Baseband  M=2^b(offset+8)  OutType=Bit  Dec=Gray  PowType=Average Power  MinDist=2  AvgPow=1  PeakPow=1  Ph=0  numSamp=1
  Rectangular QAM Demodulator Baseband9 : commdigbbndam2/Rectangular QAM Demodulator Baseband  M=2^b(offset+9)  OutType=Bit  Dec=Gray  PowType=Average Power  MinDist=2  AvgPow=1  PeakPow=1  Ph=0  numSamp=1
  Out1 : Outport
  wires:
  Rectangular QAM Demodulator Baseband1/1 -> Matrix Concatenation/1
  Rectangular QAM Demodulator Baseband2/1 -> Matrix Concatenation/2
  Rectangular QAM Demodulator Baseband3/1 -> Matrix Concatenation/3
  Rectangular QAM Demodulator Baseband4/1 -> Matrix Concatenation/4
  Rectangular QAM Demodulator Baseband5/1 -> Matrix Concatenation/5
  Rectangular QAM Demodulator Baseband6/1 -> Matrix Concatenation/6
  Rectangular QAM Demodulator Baseband7/1 -> Matrix Concatenation/7
  Rectangular QAM Demodulator Baseband8/1 -> Matrix Concatenation/8
  Rectangular QAM Demodulator Baseband9/1 -> Matrix Concatenation/9
  Rectangular QAM Demodulator Baseband10/1 -> Matrix Concatenation/10
  Rectangular QAM Demodulator Baseband11/1 -> Matrix Concatenation/11
  Rectangular QAM Demodulator Baseband12/1 -> Matrix Concatenation/12
  Rectangular QAM Demodulator Baseband13/1 -> Matrix Concatenation/13
  Rectangular QAM Demodulator Baseband14/1 -> Matrix Concatenation/14
  Rectangular QAM Demodulator Baseband15/1 -> Matrix Concatenation/15
  Rectangular QAM Demodulator Baseband16/1 -> Matrix Concatenation/16
  Demux/1 -> Rectangular QAM Demodulator Baseband1/1
  Demux/2 -> Rectangular QAM Demodulator Baseband2/1
  Demux/3 -> Rectangular QAM Demodulator Baseband3/1
  Demux/4 -> Rectangular QAM Demodulator Baseband4/1
  Demux/5 -> Rectangular QAM Demodulator Baseband5/1
  Demux/6 -> Rectangular QAM Demodulator Baseband6/1
  Demux/7 -> Rectangular QAM Demodulator Baseband7/1
  Demux/8 -> Rectangular QAM Demodulator Baseband8/1
  Demux/9 -> Rectangular QAM Demodulator Baseband9/1
  Demux/10 -> Rectangular QAM Demodulator Baseband10/1
  Demux/11 -> Rectangular QAM Demodulator Baseband11/1
  Demux/12 -> Rectangular QAM Demodulator Baseband12/1
  Demux/13 -> Rectangular QAM Demodulator Baseband13/1
  Demux/14 -> Rectangular QAM Demodulator Baseband14/1
  Demux/15 -> Rectangular QAM Demodulator Baseband15/1
  Demux/16 -> Rectangular QAM Demodulator Baseband16/1
  Matrix Concatenation/1 -> Out1/1
  In1/1 -> Demux/1

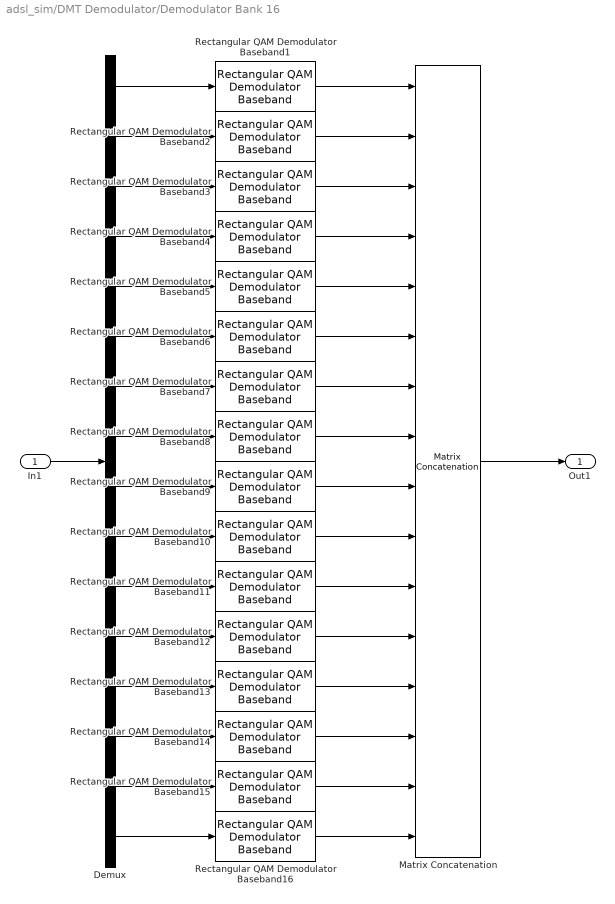
== system adsl_sim/DMT Demodulator/Demodulator Bank 16 ==
  In1 : Inport  LatchInput=off
  Demux : Demux  Outputs=16
  Matrix Concatenation : simulink/Math Operations/Matrix Concatenation  numInports=16  catMethod=Vertical
  Rectangular QAM Demodulator Baseband1 : commdigbbndam2/Rectangular QAM Demodulator Baseband  M=2^b(offset+1)  OutType=Bit  Dec=Gray  PowType=Average Power  MinDist=2  AvgPow=1  PeakPow=1  Ph=0  numSamp=1
  Rectangular QAM Demodulator Baseband10 : commdigbbndam2/Rectangular QAM Demodulator Baseband  M=2^b(offset+10)  OutType=Bit  Dec=Gray  PowType=Average Power  MinDist=2  AvgPow=1  PeakPow=1  Ph=0  numSamp=1
  Rectangular QAM Demodulator Baseband11 : commdigbbndam2/Rectangular QAM Demodulator Baseband  M=2^b(offset+11)  OutType=Bit  Dec=Gray  PowType=Average Power  MinDist=2  AvgPow=1  PeakPow=1  Ph=0  numSamp=1
  Rectangular QAM Demodulator Baseband12 : commdigbbndam2/Rectangular QAM Demodulator Baseband  M=2^b(offset+12)  OutType=Bit  Dec=Gray  PowType=Average Power  MinDist=2  AvgPow=1  PeakPow=1  Ph=0  numSamp=1
  Rectangular QAM Demodulator Baseband13 : commdigbbndam2/Rectangular QAM Demodulator Baseband  M=2^b(offset+13)  OutType=Bit  Dec=Gray  PowType=Average Power  MinDist=2  AvgPow=1  PeakPow=1  Ph=0  numSamp=1
  Rectangular QAM Demodulator Baseband14 : commdigbbndam2/Rectangular QAM Demodulator Baseband  M=2^b(offset+14)  OutType=Bit  Dec=Gray  PowType=Average Power  MinDist=2  AvgPow=1  PeakPow=1  Ph=0  numSamp=1
  Rectangular QAM Demodulator Baseband15 : commdigbbndam2/Rectangular QAM Demodulator Baseband  M=2^b(offset+15)  OutType=Bit  Dec=Gray  PowType=Average Power  MinDist=2  AvgPow=1  PeakPow=1  Ph=0  numSamp=1
  Rectangular QAM Demodulator Baseband16 : commdigbbndam2/Rectangular QAM Demodulator Baseband  M=2^b(offset+16)  OutType=Bit  Dec=Gray  PowType=Average Power  MinDist=2  AvgPow=1  PeakPow=1  Ph=0  numSamp=1
  Rectangular QAM Demodulator Baseband2 : commdigbbndam2/Rectangular QAM Demodulator Baseband  M=2^b(offset+2)  OutType=Bit  Dec=Gray  PowType=Average Power  MinDist=2  AvgPow=1  PeakPow=1  Ph=0  numSamp=1
  Rectangular QAM Demodulator Baseband3 : commdigbbndam2/Rectangular QAM Demodulator Baseband  M=2^b(offset+3)  OutType=Bit  Dec=Gray  PowType=Average Power  MinDist=2  AvgPow=1  PeakPow=1  Ph=0  numSamp=1
  Rectangular QAM Demodulator Baseband4 : commdigbbndam2/Rectangular QAM Demodulator Baseband  M=2^b(offset+4)  OutType=Bit  Dec=Gray  PowType=Average Power  MinDist=2  AvgPow=1  PeakPow=1  Ph=0  numSamp=1
  Rectangular QAM Demodulator Baseband5 : commdigbbndam2/Rectangular QAM Demodulator Baseband  M=2^b(offset+5)  OutType=Bit  Dec=Gray  PowType=Average Power  MinDist=2  AvgPow=1  PeakPow=1  Ph=0  numSamp=1
  Rectangular QAM Demodulator Baseband6 : commdigbbndam2/Rectangular QAM Demodulator Baseband  M=2^b(offset+6)  OutType=Bit  Dec=Gray  PowType=Average Power  MinDist=2  AvgPow=1  PeakPow=1  Ph=0  numSamp=1
  Rectangular QAM Demodulator Baseband7 : commdigbbndam2/Rectangular QAM Demodulator Baseband  M=2^b(offset+7)  OutType=Bit  Dec=Gray  PowType=Average Power  MinDist=2  AvgPow=1  PeakPow=1  Ph=0  numSamp=1
  Rectangular QAM Demodulator Baseband8 : commdigbbndam2/Rectangular QAM Demodulator Baseband  M=2^b(offset+8)  OutType=Bit  Dec=Gray  PowType=Average Power  MinDist=2  AvgPow=1  PeakPow=1  Ph=0  numSamp=1
  Rectangular QAM Demodulator Baseband9 : commdigbbndam2/Rectangular QAM Demodulator Baseband  M=2^b(offset+9)  OutType=Bit  Dec=Gray  PowType=Average Power  MinDist=2  AvgPow=1  PeakPow=1  Ph=0  numSamp=1
  Out1 : Outport
  wires:
  In1/1 -> Demux/1
  Matrix Concatenation/1 -> Out1/1
  Demux/16 -> Rectangular QAM Demodulator Baseband16/1
  Demux/15 -> Rectangular QAM Demodulator Baseband15/1
  Demux/14 -> Rectangular QAM Demodulator Baseband14/1
  Demux/13 -> Rectangular QAM Demodulator Baseband13/1
  Demux/12 -> Rectangular QAM Demodulator Baseband12/1
  Demux/11 -> Rectangular QAM Demodulator Baseband11/1
  Demux/10 -> Rectangular QAM Demodulator Baseband10/1
  Demux/9 -> Rectangular QAM Demodulator Baseband9/1
  Demux/8 -> Rectangular QAM Demodulator Baseband8/1
  Demux/7 -> Rectangular QAM Demodulator Baseband7/1
  Demux/6 -> Rectangular QAM Demodulator Baseband6/1
  Demux/5 -> Rectangular QAM Demodulator Baseband5/1
  Demux/4 -> Rectangular QAM Demodulator Baseband4/1
  Demux/3 -> Rectangular QAM Demodulator Baseband3/1
  Demux/2 -> Rectangular QAM Demodulator Baseband2/1
  Demux/1 -> Rectangular QAM Demodulator Baseband1/1
  Rectangular QAM Demodulator Baseband16/1 -> Matrix Concatenation/16
  Rectangular QAM Demodulator Baseband15/1 -> Matrix Concatenation/15
  Rectangular QAM Demodulator Baseband14/1 -> Matrix Concatenation/14
  Rectangular QAM Demodulator Baseband13/1 -> Matrix Concatenation/13
  Rectangular QAM Demodulator Baseband12/1 -> Matrix Concatenation/12
  Rectangular QAM Demodulator Baseband11/1 -> Matrix Concatenation/11
  Rectangular QAM Demodulator Baseband10/1 -> Matrix Concatenation/10
  Rectangular QAM Demodulator Baseband9/1 -> Matrix Concatenation/9
  Rectangular QAM Demodulator Baseband8/1 -> Matrix Concatenation/8
  Rectangular QAM Demodulator Baseband7/1 -> Matrix Concatenation/7
  Rectangular QAM Demodulator Baseband6/1 -> Matrix Concatenation/6
  Rectangular QAM Demodulator Baseband5/1 -> Matrix Concatenation/5
  Rectangular QAM Demodulator Baseband4/1 -> Matrix Concatenation/4
  Rectangular QAM Demodulator Baseband3/1 -> Matrix Concatenation/3
  Rectangular QAM Demodulator Baseband2/1 -> Matrix Concatenation/2
  Rectangular QAM Demodulator Baseband1/1 -> Matrix Concatenation/1

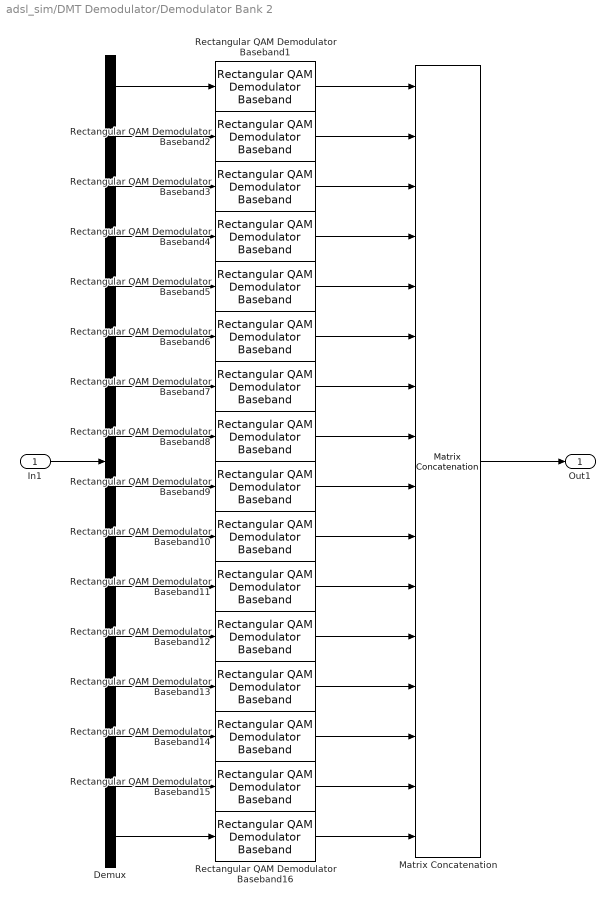
== system adsl_sim/DMT Demodulator/Demodulator Bank 2 ==
  In1 : Inport  LatchInput=off
  Demux : Demux  Outputs=16
  Matrix Concatenation : simulink/Math Operations/Matrix Concatenation  numInports=16  catMethod=Vertical
  Rectangular QAM Demodulator Baseband1 : commdigbbndam2/Rectangular QAM Demodulator Baseband  M=2^b(offset+1)  OutType=Bit  Dec=Gray  PowType=Average Power  MinDist=2  AvgPow=1  PeakPow=1  Ph=0  numSamp=1
  Rectangular QAM Demodulator Baseband10 : commdigbbndam2/Rectangular QAM Demodulator Baseband  M=2^b(offset+10)  OutType=Bit  Dec=Gray  PowType=Average Power  MinDist=2  AvgPow=1  PeakPow=1  Ph=0  numSamp=1
  Rectangular QAM Demodulator Baseband11 : commdigbbndam2/Rectangular QAM Demodulator Baseband  M=2^b(offset+11)  OutType=Bit  Dec=Gray  PowType=Average Power  MinDist=2  AvgPow=1  PeakPow=1  Ph=0  numSamp=1
  Rectangular QAM Demodulator Baseband12 : commdigbbndam2/Rectangular QAM Demodulator Baseband  M=2^b(offset+12)  OutType=Bit  Dec=Gray  PowType=Average Power  MinDist=2  AvgPow=1  PeakPow=1  Ph=0  numSamp=1
  Rectangular QAM Demodulator Baseband13 : commdigbbndam2/Rectangular QAM Demodulator Baseband  M=2^b(offset+13)  OutType=Bit  Dec=Gray  PowType=Average Power  MinDist=2  AvgPow=1  PeakPow=1  Ph=0  numSamp=1
  Rectangular QAM Demodulator Baseband14 : commdigbbndam2/Rectangular QAM Demodulator Baseband  M=2^b(offset+14)  OutType=Bit  Dec=Gray  PowType=Average Power  MinDist=2  AvgPow=1  PeakPow=1  Ph=0  numSamp=1
  Rectangular QAM Demodulator Baseband15 : commdigbbndam2/Rectangular QAM Demodulator Baseband  M=2^b(offset+15)  OutType=Bit  Dec=Gray  PowType=Average Power  MinDist=2  AvgPow=1  PeakPow=1  Ph=0  numSamp=1
  Rectangular QAM Demodulator Baseband16 : commdigbbndam2/Rectangular QAM Demodulator Baseband  M=2^b(offset+16)  OutType=Bit  Dec=Gray  PowType=Average Power  MinDist=2  AvgPow=1  PeakPow=1  Ph=0  numSamp=1
  Rectangular QAM Demodulator Baseband2 : commdigbbndam2/Rectangular QAM Demodulator Baseband  M=2^b(offset+2)  OutType=Bit  Dec=Gray  PowType=Average Power  MinDist=2  AvgPow=1  PeakPow=1  Ph=0  numSamp=1
  Rectangular QAM Demodulator Baseband3 : commdigbbndam2/Rectangular QAM Demodulator Baseband  M=2^b(offset+3)  OutType=Bit  Dec=Gray  PowType=Average Power  MinDist=2  AvgPow=1  PeakPow=1  Ph=0  numSamp=1
  Rectangular QAM Demodulator Baseband4 : commdigbbndam2/Rectangular QAM Demodulator Baseband  M=2^b(offset+4)  OutType=Bit  Dec=Gray  PowType=Average Power  MinDist=2  AvgPow=1  PeakPow=1  Ph=0  numSamp=1
  Rectangular QAM Demodulator Baseband5 : commdigbbndam2/Rectangular QAM Demodulator Baseband  M=2^b(offset+5)  OutType=Bit  Dec=Gray  PowType=Average Power  MinDist=2  AvgPow=1  PeakPow=1  Ph=0  numSamp=1
  Rectangular QAM Demodulator Baseband6 : commdigbbndam2/Rectangular QAM Demodulator Baseband  M=2^b(offset+6)  OutType=Bit  Dec=Gray  PowType=Average Power  MinDist=2  AvgPow=1  PeakPow=1  Ph=0  numSamp=1
  Rectangular QAM Demodulator Baseband7 : commdigbbndam2/Rectangular QAM Demodulator Baseband  M=2^b(offset+7)  OutType=Bit  Dec=Gray  PowType=Average Power  MinDist=2  AvgPow=1  PeakPow=1  Ph=0  numSamp=1
  Rectangular QAM Demodulator Baseband8 : commdigbbndam2/Rectangular QAM Demodulator Baseband  M=2^b(offset+8)  OutType=Bit  Dec=Gray  PowType=Average Power  MinDist=2  AvgPow=1  PeakPow=1  Ph=0  numSamp=1
  Rectangular QAM Demodulator Baseband9 : commdigbbndam2/Rectangular QAM Demodulator Baseband  M=2^b(offset+9)  OutType=Bit  Dec=Gray  PowType=Average Power  MinDist=2  AvgPow=1  PeakPow=1  Ph=0  numSamp=1
  Out1 : Outport
  wires:
  Rectangular QAM Demodulator Baseband1/1 -> Matrix Concatenation/1
  Rectangular QAM Demodulator Baseband2/1 -> Matrix Concatenation/2
  Rectangular QAM Demodulator Baseband3/1 -> Matrix Concatenation/3
  Rectangular QAM Demodulator Baseband4/1 -> Matrix Concatenation/4
  Rectangular QAM Demodulator Baseband5/1 -> Matrix Concatenation/5
  Rectangular QAM Demodulator Baseband6/1 -> Matrix Concatenation/6
  Rectangular QAM Demodulator Baseband7/1 -> Matrix Concatenation/7
  Rectangular QAM Demodulator Baseband8/1 -> Matrix Concatenation/8
  Rectangular QAM Demodulator Baseband9/1 -> Matrix Concatenation/9
  Rectangular QAM Demodulator Baseband10/1 -> Matrix Concatenation/10
  Rectangular QAM Demodulator Baseband11/1 -> Matrix Concatenation/11
  Rectangular QAM Demodulator Baseband12/1 -> Matrix Concatenation/12
  Rectangular QAM Demodulator Baseband13/1 -> Matrix Concatenation/13
  Rectangular QAM Demodulator Baseband14/1 -> Matrix Concatenation/14
  Rectangular QAM Demodulator Baseband15/1 -> Matrix Concatenation/15
  Rectangular QAM Demodulator Baseband16/1 -> Matrix Concatenation/16
  Demux/1 -> Rectangular QAM Demodulator Baseband1/1
  Demux/2 -> Rectangular QAM Demodulator Baseband2/1
  Demux/3 -> Rectangular QAM Demodulator Baseband3/1
  Demux/4 -> Rectangular QAM Demodulator Baseband4/1
  Demux/5 -> Rectangular QAM Demodulator Baseband5/1
  Demux/6 -> Rectangular QAM Demodulator Baseband6/1
  Demux/7 -> Rectangular QAM Demodulator Baseband7/1
  Demux/8 -> Rectangular QAM Demodulator Baseband8/1
  Demux/9 -> Rectangular QAM Demodulator Baseband9/1
  Demux/10 -> Rectangular QAM Demodulator Baseband10/1
  Demux/11 -> Rectangular QAM Demodulator Baseband11/1
  Demux/12 -> Rectangular QAM Demodulator Baseband12/1
  Demux/13 -> Rectangular QAM Demodulator Baseband13/1
  Demux/14 -> Rectangular QAM Demodulator Baseband14/1
  Demux/15 -> Rectangular QAM Demodulator Baseband15/1
  Demux/16 -> Rectangular QAM Demodulator Baseband16/1
  Matrix Concatenation/1 -> Out1/1
  In1/1 -> Demux/1

== system adsl_sim/DMT Demodulator/Demodulator Bank 3 ==
  In1 : Inport  LatchInput=off
  Demux : Demux  Outputs=16
  Matrix Concatenation : simulink/Math Operations/Matrix Concatenation  numInports=16  catMethod=Vertical
  Rectangular QAM Demodulator Baseband1 : commdigbbndam2/Rectangular QAM Demodulator Baseband  M=2^b(offset+1)  OutType=Bit  Dec=Gray  PowType=Average Power  MinDist=2  AvgPow=1  PeakPow=1  Ph=0  numSamp=1
  Rectangular QAM Demodulator Baseband10 : commdigbbndam2/Rectangular QAM Demodulator Baseband  M=2^b(offset+10)  OutType=Bit  Dec=Gray  PowType=Average Power  MinDist=2  AvgPow=1  PeakPow=1  Ph=0  numSamp=1
  Rectangular QAM Demodulator Baseband11 : commdigbbndam2/Rectangular QAM Demodulator Baseband  M=2^b(offset+11)  OutType=Bit  Dec=Gray  PowType=Average Power  MinDist=2  AvgPow=1  PeakPow=1  Ph=0  numSamp=1
  Rectangular QAM Demodulator Baseband12 : commdigbbndam2/Rectangular QAM Demodulator Baseband  M=2^b(offset+12)  OutType=Bit  Dec=Gray  PowType=Average Power  MinDist=2  AvgPow=1  PeakPow=1  Ph=0  numSamp=1
  Rectangular QAM Demodulator Baseband13 : commdigbbndam2/Rectangular QAM Demodulator Baseband  M=2^b(offset+13)  OutType=Bit  Dec=Gray  PowType=Average Power  MinDist=2  AvgPow=1  PeakPow=1  Ph=0  numSamp=1
  Rectangular QAM Demodulator Baseband14 : commdigbbndam2/Rectangular QAM Demodulator Baseband  M=2^b(offset+14)  OutType=Bit  Dec=Gray  PowType=Average Power  MinDist=2  AvgPow=1  PeakPow=1  Ph=0  numSamp=1
  Rectangular QAM Demodulator Baseband15 : commdigbbndam2/Rectangular QAM Demodulator Baseband  M=2^b(offset+15)  OutType=Bit  Dec=Gray  PowType=Average Power  MinDist=2  AvgPow=1  PeakPow=1  Ph=0  numSamp=1
  Rectangular QAM Demodulator Baseband16 : commdigbbndam2/Rectangular QAM Demodulator Baseband  M=2^b(offset+16)  OutType=Bit  Dec=Gray  PowType=Average Power  MinDist=2  AvgPow=1  PeakPow=1  Ph=0  numSamp=1
  Rectangular QAM Demodulator Baseband2 : commdigbbndam2/Rectangular QAM Demodulator Baseband  M=2^b(offset+2)  OutType=Bit  Dec=Gray  PowType=Average Power  MinDist=2  AvgPow=1  PeakPow=1  Ph=0  numSamp=1
  Rectangular QAM Demodulator Baseband3 : commdigbbndam2/Rectangular QAM Demodulator Baseband  M=2^b(offset+3)  OutType=Bit  Dec=Gray  PowType=Average Power  MinDist=2  AvgPow=1  PeakPow=1  Ph=0  numSamp=1
  Rectangular QAM Demodulator Baseband4 : commdigbbndam2/Rectangular QAM Demodulator Baseband  M=2^b(offset+4)  OutType=Bit  Dec=Gray  PowType=Average Power  MinDist=2  AvgPow=1  PeakPow=1  Ph=0  numSamp=1
  Rectangular QAM Demodulator Baseband5 : commdigbbndam2/Rectangular QAM Demodulator Baseband  M=2^b(offset+5)  OutType=Bit  Dec=Gray  PowType=Average Power  MinDist=2  AvgPow=1  PeakPow=1  Ph=0  numSamp=1
  Rectangular QAM Demodulator Baseband6 : commdigbbndam2/Rectangular QAM Demodulator Baseband  M=2^b(offset+6)  OutType=Bit  Dec=Gray  PowType=Average Power  MinDist=2  AvgPow=1  PeakPow=1  Ph=0  numSamp=1
  Rectangular QAM Demodulator Baseband7 : commdigbbndam2/Rectangular QAM Demodulator Baseband  M=2^b(offset+7)  OutType=Bit  Dec=Gray  PowType=Average Power  MinDist=2  AvgPow=1  PeakPow=1  Ph=0  numSamp=1
  Rectangular QAM Demodulator Baseband8 : commdigbbndam2/Rectangular QAM Demodulator Baseband  M=2^b(offset+8)  OutType=Bit  Dec=Gray  PowType=Average Power  MinDist=2  AvgPow=1  PeakPow=1  Ph=0  numSamp=1
  Rectangular QAM Demodulator Baseband9 : commdigbbndam2/Rectangular QAM Demodulator Baseband  M=2^b(offset+9)  OutType=Bit  Dec=Gray  PowType=Average Power  MinDist=2  AvgPow=1  PeakPow=1  Ph=0  numSamp=1
  Out1 : Outport
  wires:
  Rectangular QAM Demodulator Baseband1/1 -> Matrix Concatenation/1
  Rectangular QAM Demodulator Baseband2/1 -> Matrix Concatenation/2
  Rectangular QAM Demodulator Baseband3/1 -> Matrix Concatenation/3
  Rectangular QAM Demodulator Baseband4/1 -> Matrix Concatenation/4
  Rectangular QAM Demodulator Baseband5/1 -> Matrix Concatenation/5
  Rectangular QAM Demodulator Baseband6/1 -> Matrix Concatenation/6
  Rectangular QAM Demodulator Baseband7/1 -> Matrix Concatenation/7
  Rectangular QAM Demodulator Baseband8/1 -> Matrix Concatenation/8
  Rectangular QAM Demodulator Baseband9/1 -> Matrix Concatenation/9
  Rectangular QAM Demodulator Baseband10/1 -> Matrix Concatenation/10
  Rectangular QAM Demodulator Baseband11/1 -> Matrix Concatenation/11
  Rectangular QAM Demodulator Baseband12/1 -> Matrix Concatenation/12
  Rectangular QAM Demodulator Baseband13/1 -> Matrix Concatenation/13
  Rectangular QAM Demodulator Baseband14/1 -> Matrix Concatenation/14
  Rectangular QAM Demodulator Baseband15/1 -> Matrix Concatenation/15
  Rectangular QAM Demodulator Baseband16/1 -> Matrix Concatenation/16
  Demux/1 -> Rectangular QAM Demodulator Baseband1/1
  Demux/2 -> Rectangular QAM Demodulator Baseband2/1
  Demux/3 -> Rectangular QAM Demodulator Baseband3/1
  Demux/4 -> Rectangular QAM Demodulator Baseband4/1
  Demux/5 -> Rectangular QAM Demodulator Baseband5/1
  Demux/6 -> Rectangular QAM Demodulator Baseband6/1
  Demux/7 -> Rectangular QAM Demodulator Baseband7/1
  Demux/8 -> Rectangular QAM Demodulator Baseband8/1
  Demux/9 -> Rectangular QAM Demodulator Baseband9/1
  Demux/10 -> Rectangular QAM Demodulator Baseband10/1
  Demux/11 -> Rectangular QAM Demodulator Baseband11/1
  Demux/12 -> Rectangular QAM Demodulator Baseband12/1
  Demux/13 -> Rectangular QAM Demodulator Baseband13/1
  Demux/14 -> Rectangular QAM Demodulator Baseband14/1
  Demux/15 -> Rectangular QAM Demodulator Baseband15/1
  Demux/16 -> Rectangular QAM Demodulator Baseband16/1
  Matrix Concatenation/1 -> Out1/1
  In1/1 -> Demux/1
